simulink model "simu_repaso"  (R2021a)
settings: Solver=ode4  StartTime=0.0  StopTime=2000  FixedStep=0.01  RelTol=1e-3
values from neighbouring files (symbols this model uses):
  A = double( subs( jacobian(hdot, h), [h u], [h0 u0] ) )    [script_repaso.m]
  B = double( subs( jacobian(hdot, u), [h u], [h0 u0] ) )    [script_repaso.m]
  C = 1    [script_repaso.m]
  h0 = double(h0)    [script_repaso.m]
  Qi = double(Qi)    [script_repaso.m]
  u0 = double(u0)    [script_repaso.m]
libraries: cstblocks x5
settings Model: Creator=frand  LastModifiedBy=frand

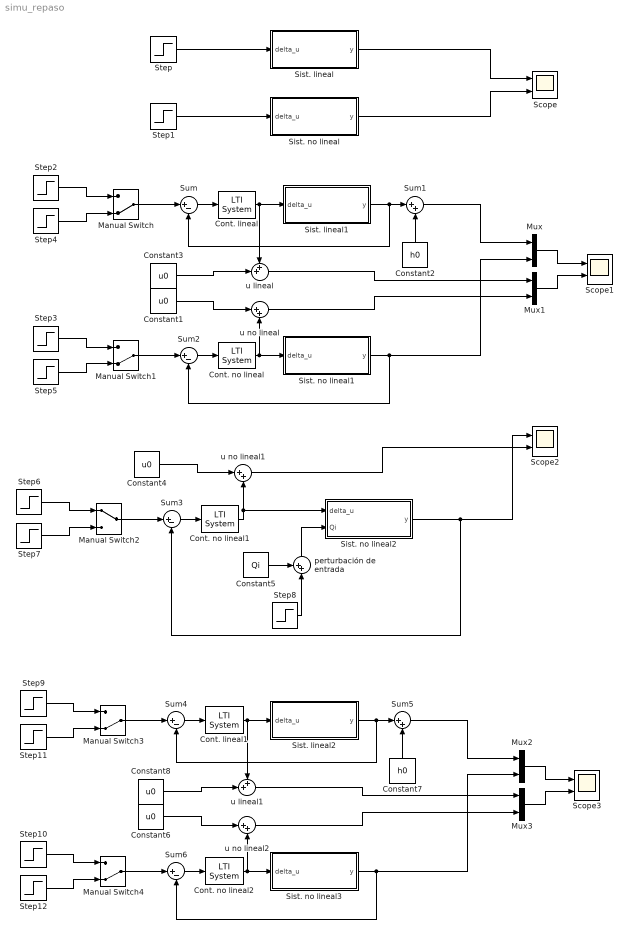
== system simu_repaso ==
  Constant{1,3..4,6,8} (5 alike) : Constant  Value=u0
  Constant2 : Constant  Value=h0
  Constant5 : Constant  Value=Qi
  Constant7 : Constant  Value=h0
  Cont. lineal : cstblocks/LTI System  sys=Cont  IC=[]
  Cont. lineal1 : cstblocks/LTI System  sys=C  IC=[]
  Cont. no lineal : cstblocks/LTI System  sys=C  IC=[]
  Cont. no lineal1 : cstblocks/LTI System  sys=C  IC=[]
  Cont. no lineal2 : cstblocks/LTI System  sys=C  IC=[]
  Manual Switch{,1,3..4} (4 alike) : ManualSwitch  CurrentSetting=0
  Manual Switch2 : ManualSwitch
  Mux{,1..3} (4 alike) : Mux  Inputs=2
  Scope{,1..3} (4 alike) : Scope  NumInputPorts=2
  Sist. lineal : Subsystem
  Sist. lineal1 : Subsystem
  Sist. lineal2 : Subsystem
  Sist. no lineal : Subsystem
  Sist. no lineal1 : Subsystem
  Sist. no lineal2 : Subsystem
  Sist. no lineal3 : Subsystem
  Step : Step  After=.1*u0  SampleTime=0
  Step1 : Step  After=.1*u0  SampleTime=0
  Step10 : Step  Before=.45  After=.35  SampleTime=0
  Step11 : Step  After=.1  SampleTime=0
  Step12 : Step  Before=.45  After=.55  SampleTime=0
  Step2 : Step  After=-.1  SampleTime=0
  Step3 : Step  Before=.45  After=.35  SampleTime=0
  Step4 : Step  After=.1  SampleTime=0
  Step5 : Step  Before=.45  After=.55  SampleTime=0
  Step6 : Step  Before=.45  After=.35  SampleTime=0
  Step7 : Step  Before=.45  After=.55  SampleTime=0
  Step8 : Step  After=-0.1*Qi  SampleTime=500
  Step9 : Step  After=-.1  SampleTime=0
  Sum{,2..4,6} (5 alike) : Sum  Inputs=|+-
  Sum1 : Sum  Inputs=|++
  Sum5 : Sum  Inputs=|++
  perturbación de entrada : Sum  Inputs=++|
  u lineal : Sum  Inputs=++|
  u lineal1 : Sum  Inputs=++|
  u no lineal : Sum  Inputs=|++
  u no lineal1 : Sum  Inputs=|++
  u no lineal2 : Sum  Inputs=|++
  wires:
  Step/1 -> Sist. lineal/1(delta_u)
  Sist. lineal/1(y) -> Scope/1
  Step1/1 -> Sist. no lineal/1(delta_u)
  Sist. no lineal/1(y) -> Scope/2
  Sist. no lineal1/1(y) -> Mux/2, Sum2/2
  Sist. lineal1/1(y) -> Sum1/1, Sum/2
  Cont. lineal/1 -> u lineal/1, Sist. lineal1/1(delta_u)
  Sum/1 -> Cont. lineal/1
  Sum1/1 -> Mux/1
  Constant2/1 -> Sum1/2
  Cont. no lineal/1 -> u no lineal/2, Sist. no lineal1/1(delta_u)
  Sum2/1 -> Cont. no lineal/1
  Mux1/1 -> Scope1/2
  Mux/1 -> Scope1/1
  Constant1/1 -> u no lineal/1
  u no lineal/1 -> Mux1/2
  u lineal/1 -> Mux1/1
  Constant3/1 -> u lineal/2
  Step2/1 -> Manual Switch/1
  Step4/1 -> Manual Switch/2
  Manual Switch/1 -> Sum/1
  Manual Switch1/1 -> Sum2/1
  Step5/1 -> Manual Switch1/2
  Step3/1 -> Manual Switch1/1
  Step6/1 -> Manual Switch2/1
  Step7/1 -> Manual Switch2/2
  Manual Switch2/1 -> Sum3/1
  u no lineal1/1 -> Scope2/2
  Constant4/1 -> u no lineal1/1
  Sum3/1 -> Cont. no lineal1/1
  Cont. no lineal1/1 -> Sist. no lineal2/1(delta_u), u no lineal1/2
  Sist. no lineal2/1(y) -> Scope2/1, Sum3/2
  perturbación de entrada/1 -> Sist. no lineal2/2(Qi)
  Constant5/1 -> perturbación de entrada/1
  Step8/1 -> perturbación de entrada/2
  Step10/1 -> Manual Switch4/1
  Step12/1 -> Manual Switch4/2
  Manual Switch4/1 -> Sum6/1
  Manual Switch3/1 -> Sum4/1
  Step11/1 -> Manual Switch3/2
  Step9/1 -> Manual Switch3/1
  Constant8/1 -> u lineal1/2
  u lineal1/1 -> Mux3/1
  u no lineal2/1 -> Mux3/2
  Constant6/1 -> u no lineal2/1
  Mux2/1 -> Scope3/1
  Mux3/1 -> Scope3/2
  Sum6/1 -> Cont. no lineal2/1
  Cont. no lineal2/1 -> Sist. no lineal3/1(delta_u), u no lineal2/2
  Constant7/1 -> Sum5/2
  Sum5/1 -> Mux2/1
  Sum4/1 -> Cont. lineal1/1
  Cont. lineal1/1 -> Sist. lineal2/1(delta_u), u lineal1/1
  Sist. lineal2/1(y) -> Sum4/2, Sum5/1
  Sist. no lineal3/1(y) -> Sum6/2, Mux2/2

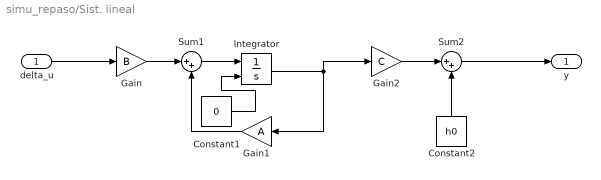
== system simu_repaso/Sist. lineal ==
  delta_u : Inport
  Constant1 : Constant  Value=0
  Constant2 : Constant  Value=h0
  Gain : Gain  Gain=B
  Gain1 : Gain  Gain=A
  Gain2 : Gain  Gain=C
  Integrator : Integrator  InitialConditionSource=external
  Sum1 : Sum  Inputs=|++
  Sum2 : Sum  Inputs=|++
  y : Outport
  wires:
  Sum2/1 -> y/1
  Gain/1 -> Sum1/1
  Sum1/1 -> Integrator/1
  Gain1/1 -> Sum1/2
  Constant2/1 -> Sum2/2
  Gain2/1 -> Sum2/1
  delta_u/1 -> Gain/1
  Integrator/1 -> Gain2/1, Gain1/1
  Constant1/1 -> Integrator/2

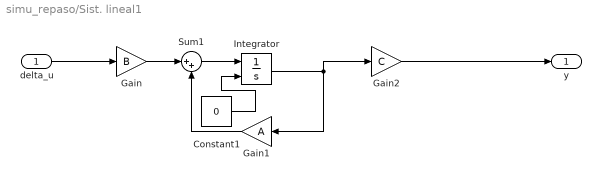
== system simu_repaso/Sist. lineal1 ==
  delta_u : Inport
  Constant1 : Constant  Value=0
  Gain : Gain  Gain=B
  Gain1 : Gain  Gain=A
  Gain2 : Gain  Gain=C
  Integrator : Integrator  InitialConditionSource=external
  Sum1 : Sum  Inputs=|++
  y : Outport
  wires:
  Constant1/1 -> Integrator/2
  Integrator/1 -> Gain1/1, Gain2/1
  delta_u/1 -> Gain/1
  Gain1/1 -> Sum1/2
  Sum1/1 -> Integrator/1
  Gain/1 -> Sum1/1
  Gain2/1 -> y/1

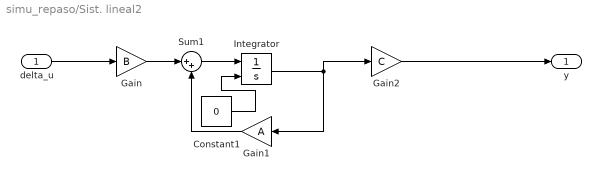
== system simu_repaso/Sist. lineal2 ==
  delta_u : Inport
  Constant1 : Constant  Value=0
  Gain : Gain  Gain=B
  Gain1 : Gain  Gain=A
  Gain2 : Gain  Gain=C
  Integrator : Integrator  InitialConditionSource=external
  Sum1 : Sum  Inputs=|++
  y : Outport
  wires:
  Gain2/1 -> y/1
  Gain/1 -> Sum1/1
  Sum1/1 -> Integrator/1
  Gain1/1 -> Sum1/2
  delta_u/1 -> Gain/1
  Integrator/1 -> Gain2/1, Gain1/1
  Constant1/1 -> Integrator/2

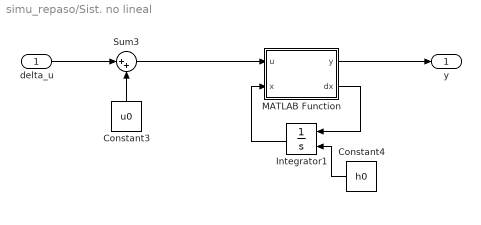
== system simu_repaso/Sist. no lineal ==
  delta_u : Inport
  Constant3 : Constant  Value=u0
  Constant4 : Constant  Value=h0
  Integrator1 : Integrator  InitialConditionSource=external
  MATLAB Function : MATLAB Function  TreatAsAtomicUnit=on
  Sum3 : Sum  Inputs=|++
  y : Outport
  wires:
  MATLAB Function/1(y) -> y/1
  Constant3/1 -> Sum3/2
  MATLAB Function/2(dx) -> Integrator1/1
  Sum3/1 -> MATLAB Function/1(u)
  delta_u/1 -> Sum3/1
  Integrator1/1 -> MATLAB Function/2(x)
  Constant4/1 -> Integrator1/2

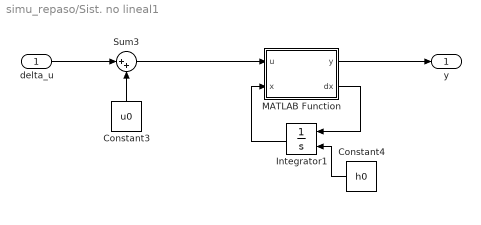
== system simu_repaso/Sist. no lineal1 ==
  delta_u : Inport
  Constant3 : Constant  Value=u0
  Constant4 : Constant  Value=h0
  Integrator1 : Integrator  InitialConditionSource=external
  MATLAB Function : MATLAB Function  TreatAsAtomicUnit=on
  Sum3 : Sum  Inputs=|++
  y : Outport
  wires:
  Constant4/1 -> Integrator1/2
  Integrator1/1 -> MATLAB Function/2(x)
  delta_u/1 -> Sum3/1
  Sum3/1 -> MATLAB Function/1(u)
  MATLAB Function/2(dx) -> Integrator1/1
  Constant3/1 -> Sum3/2
  MATLAB Function/1(y) -> y/1

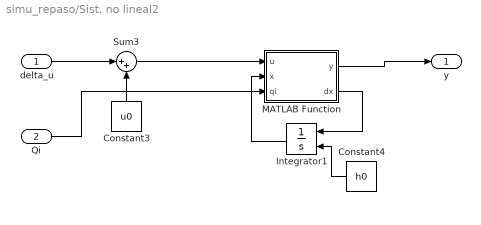
== system simu_repaso/Sist. no lineal2 ==
  delta_u : Inport
  Qi : Inport  Port=2
  Constant3 : Constant  Value=u0
  Constant4 : Constant  Value=h0
  Integrator1 : Integrator  InitialConditionSource=external
  MATLAB Function : MATLAB Function  TreatAsAtomicUnit=on
  Sum3 : Sum  Inputs=|++
  y : Outport
  wires:
  MATLAB Function/1(y) -> y/1
  Constant3/1 -> Sum3/2
  MATLAB Function/2(dx) -> Integrator1/1
  Sum3/1 -> MATLAB Function/1(u)
  delta_u/1 -> Sum3/1
  Integrator1/1 -> MATLAB Function/2(x)
  Constant4/1 -> Integrator1/2
  Qi/1 -> MATLAB Function/3(qi)

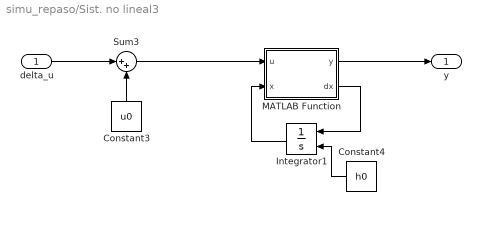
== system simu_repaso/Sist. no lineal3 ==
  delta_u : Inport
  Constant3 : Constant  Value=u0
  Constant4 : Constant  Value=h0
  Integrator1 : Integrator  InitialConditionSource=external
  MATLAB Function : MATLAB Function  TreatAsAtomicUnit=on
  Sum3 : Sum  Inputs=|++
  y : Outport
  wires:
  MATLAB Function/1(y) -> y/1
  Constant3/1 -> Sum3/2
  MATLAB Function/2(dx) -> Integrator1/1
  Sum3/1 -> MATLAB Function/1(u)
  delta_u/1 -> Sum3/1
  Integrator1/1 -> MATLAB Function/2(x)
  Constant4/1 -> Integrator1/2

== matlab function simu_repaso/Sist. no lineal/MATLAB Function ==
  data: u input; y output; x input; dx output
function [y ,dx] = fcn(u, x)

dx = (3.75e-8*(-9465169.035*sqrt(x)*u+3.2e6))/(100*x^2+60*x+9);
y = x;
end

== matlab function simu_repaso/Sist. no lineal1/MATLAB Function ==
  data: u input; y output; x input; dx output
function [y ,dx] = fcn(u, x)

dx = (3.75e-8*(-9465169.035*sqrt(x)*u+3.2e6))/(100*x^2+60*x+9);
y = x;
end

== matlab function simu_repaso/Sist. no lineal2/MATLAB Function ==
  data: u input; y output; x input; dx output; qi input
function [y ,dx] = fcn(u, x, qi)
d = 0.01065;
g = 9.18;
A = pi*(d/2)^2*u;
Qo = sqrt(2*g*x)*A;
Vdot = 0.11111111111111111111111111111111*x^2 + 0.066666666666666666666666666666667*x + 0.01;
dx = (qi -Qo)/Vdot;
y = x;
end

== matlab function simu_repaso/Sist. no lineal3/MATLAB Function ==
  data: u input; y output; x input; dx output
function [y ,dx] = fcn(u, x)

dx = (3.75e-8*(-9465169.035*sqrt(x)*u+3.2e6))/(100*x^2+60*x+9);
y = x;
end
